simulink model "NonLinear_Plant_D2"  (R2020b)
settings: Solver=ode3  StartTime=0.0  StopTime=10.0  FixedStep=0.001  RelTol=1e-3
undefined symbols (not defined in the file): alpha0, alpha_dot0, B, D_p, D_r, g, J_p, J_r, K_m, K_Report, L_p, L_r, m_p, R_m, theta0, theta_dot0
settings Model: Creator=Amir  LastModifiedBy=Amir

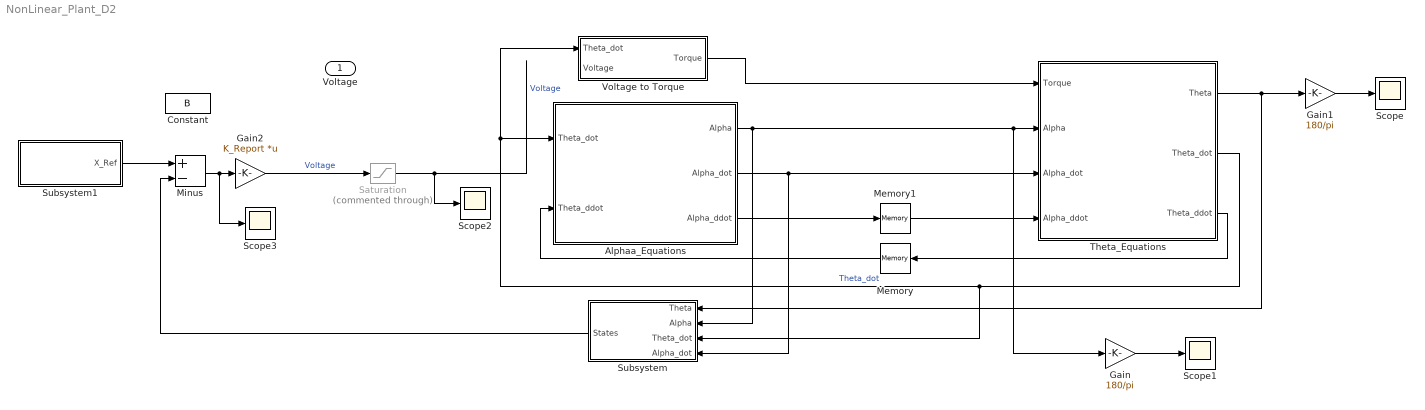
== system NonLinear_Plant_D2 ==
  Voltage : Inport
  Alphaa_Equations : Subsystem
  Constant : Constant  Value=B
  Gain : Gain  Gain=180/pi
  Gain1 : Gain  Gain=180/pi
  Gain2 : Gain  Gain=K_Report  Multiplication=Matrix(K*u)
  Memory : Memory  InheritSampleTime=on
  Memory1 : Memory  InheritSampleTime=on
  Minus : Sum  Inputs=+-
  Saturation : Saturate  Commented=through  UpperLimit=15  LowerLimit=-15
  Scope{,1..3} (4 alike) : Scope
  Subsystem : Subsystem
  Subsystem1 : Subsystem
  Theta_Equations : Subsystem
  Voltage to Torque : Subsystem
  wires:
  Saturation/1 -> Scope2/1  "Voltage"
  Theta_Equations/2(Theta_dot) -> Voltage to Torque/1(Theta_dot), Alphaa_Equations/1(Theta_dot), Subsystem/3(Theta_dot)  "Theta_dot"
  Theta_Equations/3(Theta_ddot) -> Memory/1
  Alphaa_Equations/2(Alpha_dot) -> Subsystem/4(Alpha_dot), Theta_Equations/3(Alpha_dot)
  Alphaa_Equations/3(Alpha_ddot) -> Memory1/1
  Theta_Equations/1(Theta) -> Gain1/1, Subsystem/1(Theta)
  Alphaa_Equations/1(Alpha) -> Subsystem/2(Alpha), Gain/1, Theta_Equations/2(Alpha)
  Gain/1 -> Scope1/1
  Memory/1 -> Alphaa_Equations/2(Theta_ddot)
  Memory1/1 -> Theta_Equations/4(Alpha_ddot)
  Voltage to Torque/1(Torque) -> Theta_Equations/1(Torque)
  Gain2/1 -> Saturation/1  "Voltage"
  Subsystem1/1(X_Ref) -> Minus/1
  Subsystem/1(States) -> Minus/2
  Minus/1 -> Scope3/1, Gain2/1
  Gain1/1 -> Scope/1

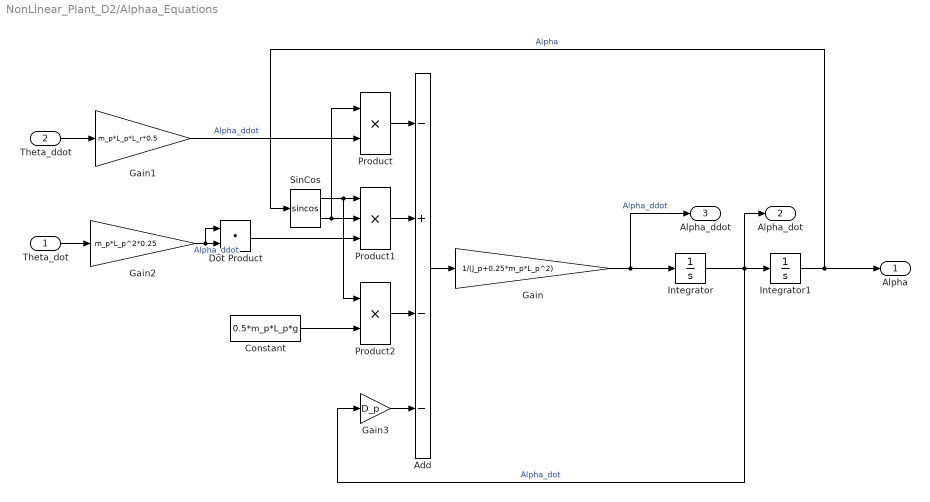
== system NonLinear_Plant_D2/Alphaa_Equations ==
  Theta_dot : Inport
  Theta_ddot : Inport  Port=2
  Add : Sum  Inputs=-+--
  Constant : Constant  Value=0.5*m_p*L_p*g
  Dot Product : DotProduct  InputSameDT=on  OutDataTypeStr=Inherit: Inherit via internal rule
  Gain : Gain  Gain=1/(J_p+0.25*m_p*L_p^2)
  Gain1 : Gain  Gain=m_p*L_p*L_r*0.5
  Gain2 : Gain  Gain=m_p*L_p^2*0.25
  Gain3 : Gain  Gain=D_p
  Integrator : Integrator  InitialCondition=alpha_dot0
  Integrator1 : Integrator  InitialCondition=alpha0
  Product : Product
  Product1 : Product  Inputs=3
  Product2 : Product
  SinCos : Trigonometry  Operator=sincos
  Alpha : Outport
  Alpha_dot : Outport  Port=2
  Alpha_ddot : Outport  Port=3
  wires:
  Gain2/1 -> Dot Product/1, Dot Product/2  "Alpha_ddot"
  Gain1/1 -> Product/2  "Alpha_ddot"
  Product/1 -> Add/1
  SinCos/1 -> Product2/1, Product1/1
  Theta_ddot/1 -> Gain1/1
  Product1/1 -> Add/2
  Gain3/1 -> Add/4
  Gain/1 -> Alpha_ddot/1, Integrator/1  "Alpha_ddot"
  Integrator/1 -> Alpha_dot/1, Gain3/1, Integrator1/1  "Alpha_dot"
  Integrator1/1 -> Alpha/1, SinCos/1  "Alpha"
  Add/1 -> Gain/1
  Dot Product/1 -> Product1/3
  Theta_dot/1 -> Gain2/1
  SinCos/2 -> Product/1, Product1/2
  Constant/1 -> Product2/2
  Product2/1 -> Add/3

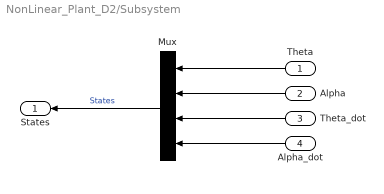
== system NonLinear_Plant_D2/Subsystem ==
  Theta : Inport
  Alpha : Inport  Port=2
  Theta_dot : Inport  Port=3
  Alpha_dot : Inport  Port=4
  Mux : Mux
  States : Outport
  wires:
  Alpha_dot/1 -> Mux/4
  Mux/1 -> States/1  "States"
  Theta_dot/1 -> Mux/3
  Theta/1 -> Mux/1
  Alpha/1 -> Mux/2

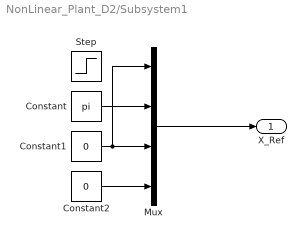
== system NonLinear_Plant_D2/Subsystem1 ==
  Constant : Constant  Value=pi
  Constant1 : Constant  Value=0
  Constant2 : Constant  Value=0
  Mux : Mux
  Step : Step  Time=2  After=pi/2  SampleTime=0
  X_Ref : Outport
  wires:
  Mux/1 -> X_Ref/1
  Constant/1 -> Mux/2
  Constant2/1 -> Mux/4
  Constant1/1 -> Mux/1, Mux/3

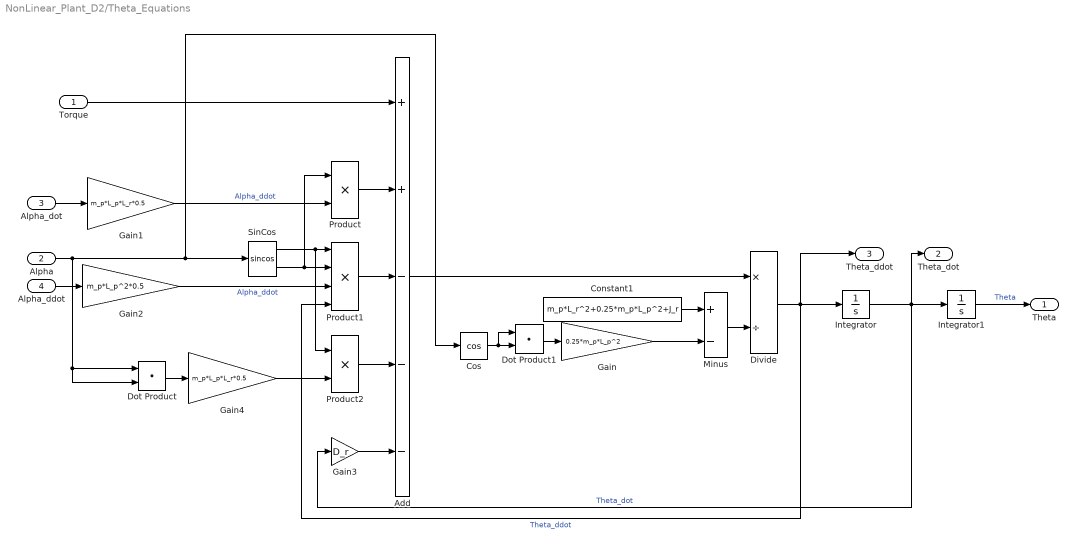
== system NonLinear_Plant_D2/Theta_Equations ==
  Torque : Inport
  Alpha : Inport  Port=2
  Alpha_dot : Inport  Port=3
  Alpha_ddot : Inport  Port=4
  Add : Sum  Inputs=++---
  Constant1 : Constant  Value=m_p*L_r^2+0.25*m_p*L_p^2+J_r
  Cos : Trigonometry  Operator=cos
  Divide : Product  Inputs=*/
  Dot Product : DotProduct  InputSameDT=on  OutDataTypeStr=Inherit: Inherit via internal rule
  Dot Product1 : DotProduct  InputSameDT=on  OutDataTypeStr=Inherit: Inherit via internal rule
  Gain : Gain  Gain=0.25*m_p*L_p^2
  Gain1 : Gain  Gain=m_p*L_p*L_r*0.5
  Gain2 : Gain  Gain=m_p*L_p^2*0.5
  Gain3 : Gain  Gain=D_r
  Gain4 : Gain  Gain=m_p*L_p*L_r*0.5
  Integrator : Integrator  InitialCondition=theta_dot0
  Integrator1 : Integrator  InitialCondition=theta0
  Minus : Sum  Inputs=+-
  Product : Product
  Product1 : Product  Inputs=4
  Product2 : Product
  SinCos : Trigonometry  Operator=sincos
  Theta : Outport
  Theta_dot : Outport  Port=2
  Theta_ddot : Outport  Port=3
  wires:
  Product2/1 -> Add/4
  Gain4/1 -> Product2/2
  SinCos/2 -> Product/1, Product1/2
  Alpha_ddot/1 -> Gain2/1
  Add/1 -> Divide/1
  Integrator1/1 -> Theta/1  "Theta"
  Integrator/1 -> Gain3/1, Integrator1/1, Theta_dot/1  "Theta_dot"
  Divide/1 -> Theta_ddot/1, Product1/4, Integrator/1  "Theta_ddot"
  Gain3/1 -> Add/5
  Product1/1 -> Add/3
  Alpha_dot/1 -> Gain1/1
  SinCos/1 -> Product2/1, Product1/1
  Product/1 -> Add/2
  Gain1/1 -> Product/2  "Alpha_ddot"
  Gain2/1 -> Product1/3  "Alpha_ddot"
  Constant1/1 -> Minus/1
  Alpha/1 -> Dot Product/2, Dot Product/1, Cos/1, SinCos/1
  Cos/1 -> Dot Product1/1, Dot Product1/2
  Dot Product1/1 -> Gain/1
  Gain/1 -> Minus/2
  Minus/1 -> Divide/2
  Torque/1 -> Add/1
  Dot Product/1 -> Gain4/1

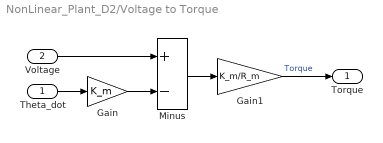
== system NonLinear_Plant_D2/Voltage to Torque ==
  Theta_dot : Inport
  Voltage : Inport  Port=2
  Gain : Gain  Gain=K_m
  Gain1 : Gain  Gain=K_m/R_m
  Minus : Sum  Inputs=+-
  Torque : Outport
  wires:
  Gain/1 -> Minus/2
  Voltage/1 -> Minus/1
  Gain1/1 -> Torque/1  "Torque"
  Minus/1 -> Gain1/1
  Theta_dot/1 -> Gain/1
